simulink model "BEVModel_Alternate"  (R2023a)
settings: Solver=VariableStepAuto  StartTime=0.0  StopTime=1  RelTol=1e-3
undefined symbols (not defined in the file or in its folder): Ion, Lithium
libraries: fl_lib x9, nesl_utility x7, ee_lib x3, autolibshared x2, spsBatteryLib x1, spsControlledCurrentSourceLib x1, sps_lib x1
settings Model: Creator=koush  LastModifiedBy=koush

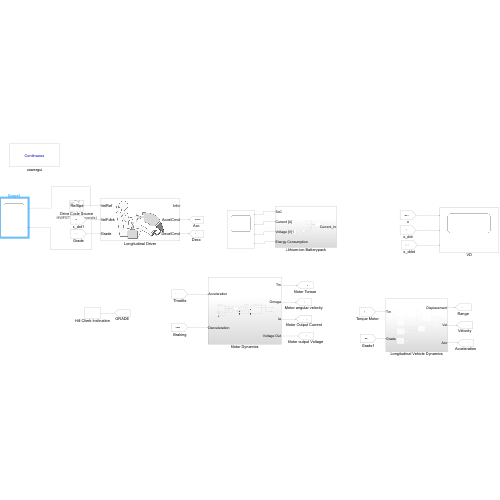
[thumbnail: Simulink's stored preview of the top-level diagram]
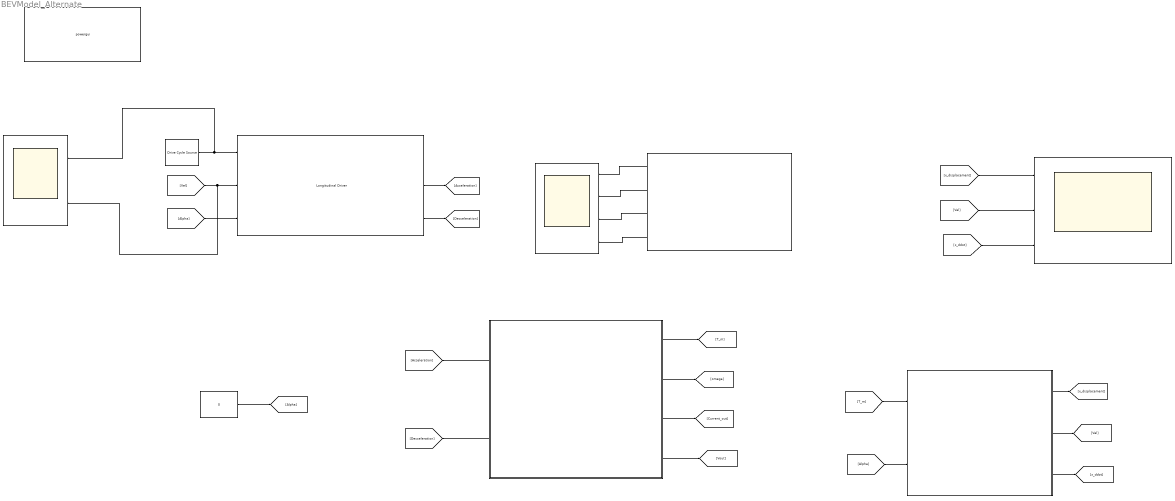
== system BEVModel_Alternate ==
  Drive Cycle Source : autolibshared/Drive Cycle Source  cycleVar=HWFET  fileVar=cycleFTP75.mat  tfinal="765  seconds"  cycleRepeat=off  outAccPort=off  outGearPort=off  gearList=No gear data  t_wot1=5  xdot_woto=0  xdot_wot1=30  t_wot2=20  xdot_wot2=0  t_wotend=30  srcUnit=m/s  outUnit=m/s  srcAccUnit=m/s/s  outAccUnit=m/s^2  dt=0  aMode=1  faultOption=off  velBnd=2  velBndUnit=mph  inUnit=m/s  timeBnd=1  failOption=off  stopSim=off  maxFaultCnt=10  maxFaultTime=2  maxTotFaultTime=15  traceOption=off  dtTrace=1  traceWindow=10  lastDCname=HWFET  lastOutUnit=mph  lastDT=0  lastTB=1  lastSB=2  forceCalcBound=off
  Hill Climb Inclination : Constant  Value=0
  Lithium-ion Batterypack : Subsystem
  Longitudinal Driver : autolibshared/Longitudinal Driver  extAccelOvr=off  extDecelOvr=off  extAccelHld=off  extDecelHld=off  extAccelZero=off  extDecelZero=off  cntrlType=PI  shftType=None  velUnits=m/s  gearOut=off  Kp=15  Ki=1  Kff=.05  Kg=.01  VehVelVec=[0 100]  KffVec=[.1 .1]  KpVec=[10 10]  KiVec=[5 5]  KgVec=[0 0]  m=1500  Kpt=3000  tau=.1  L=2  aR=200  bR=2.5  cR=.5  g=9.81  vnom=100  Kaw=.1  tauerr=.03  tauPt=2  GearInit=0  tShift=.1  pdlVec=[0.1 0.4 0.5 0.9]  upShftTbl=[-1 12.9375 26.4375 39.9375 51.18749999999999 62.4375 72.84375 83.25;-1 16.3125 29.8125 43.3125 54.5624 65.8125 76.78125 87.75;-1 19.6875 33.1875 46.68749999999999 57.9375 69.1875 80.71875 92.25;-1 33 52.5 77.25 100.5 138.75 161.875 185]  dwnShftTbl=[1 9.5625 23.0625 36.5625 47.8125 59.0625 68.90625 78.75;1 12.9375 26.4375 39.9375 51.18749999999999 62.4375 72.84375 83.25;1 16.3125 29.8125 43.3125 54.562499 65.8125 76.78125 87.75;1 19.6875 33.1875 46.68749999999999 57.9375 69.1875 80.71875 92.25]  tClutch=.5  tRev=.5  tPark=120  aMode=1  UpGearVec="[0  1  2  3  4  5  6  7]"  DownGearVec="[1  2  3  4  5  6  7  8]"
  Longitudinal Vehicle Dynamics : Subsystem
  Motor Dynamics : Subsystem
  Scope : Scope  NumInputPorts=4
  Scope1 : Scope  NumInputPorts=2
  VD : Scope  NumInputPorts=3
  powergui : sps_lib/powergui  Priority=1  SimulationMode=Continuous  SampleTime=50e-6  frequency=60  Iterations=50  frequencyindice=0  Pbase=100e6  ErrMax=1e-4  UnitsV=kV  UnitsW=MW  buscounter=0  FunctionMessages=off  echomessages=off  EnableUseOfTLC=off  CurrentSourceSwitches=off  DisableSnubberDevices=off  DisableRonSwitches=off  DisableVfSwitches=off  DisplayEquations=off  AutomaticDiscreteSolvers=off  SolverType=Tustin/Backward Euler (TBE)  Interpol=off  ExternalGateDelay=off  methode=off  Ts=100  x0status=blocks  SPID=on  SwTol=0  HookPort=off  NonlinearTolerance=1e-4  nMaxIteration=100  ContinueOnMaxIteration=off  RestoreLinks=warning  ResistiveCurrentMeasurement=off  Frange=[0:2:500]  Ylog=off  Xlog=on  ShowGrid=off  save=off  variable=ZData  structure=0  ZoomFFT=off  StartTime=0.0  cycles=1  DisplayStyle=1  fundamental=60  FreqAxis=off  MaxFrequency=1000  frequencyindicesteady=1  RmsSteady=1  display=off
  wires:
  [Vel] -> Scope1/2, Longitudinal Driver/2
  Longitudinal Driver/3 -> [Decceleration]
  [Alpha] -> Longitudinal Vehicle Dynamics/2(Grade)
  [x_displacement] -> VD/1
  Motor Dynamics/1(Tm) -> [T_m]
  [Alpha] -> Longitudinal Driver/3
  Drive Cycle Source/1 -> Scope1/1, Longitudinal Driver/1
  Longitudinal Vehicle Dynamics/1(Displacement) -> [x_displacement]
  [Vel] -> VD/2
  [x_ddot] -> VD/3
  [T_m] -> Longitudinal Vehicle Dynamics/1(Tm)
  Hill Climb Inclination/1 -> [Alpha]
  Longitudinal Vehicle Dynamics/2(Vel) -> [Vel]
  Longitudinal Driver/2 -> [Acceleration]
  Longitudinal Vehicle Dynamics/3(Acc) -> [x_ddot]
  [Acceleration] -> Motor Dynamics/1(Acceleration)
  [Decceleration] -> Motor Dynamics/2(Decceleration)
  Motor Dynamics/2(Omega) -> [omega]
  Motor Dynamics/3(Ia) -> [Current_out]
  Motor Dynamics/4(Voltage Out) -> [Vout]
  Lithium-ion Batterypack/1(SoC) -> Scope/1
  Lithium-ion Batterypack/2(Current [A]) -> Scope/2
  Lithium-ion Batterypack/3(Voltage [V]1) -> Scope/3
  Lithium-ion Batterypack/4(Energy Consumption) -> Scope/4

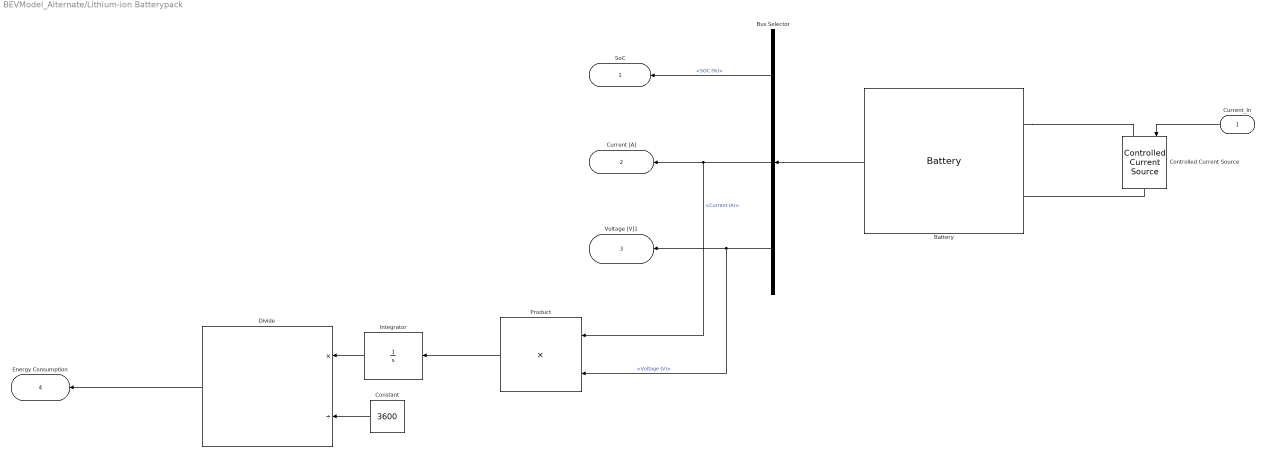
== system BEVModel_Alternate/Lithium-ion Batterypack ==
  Current_In : Inport
  Battery : spsBatteryLib/Battery  BatType=Lithium-Ion  ShowTempParam=off  ThermalPreset=no  ShowAgeParam=off  NomV=7.2  NomQ=5.4  SOC=100  Batt_Tr=30  PresetModel=on  MaxQ=5.4  MinV=5.4  FullV=8.3807  Dis_rate=2.3478  R=0.013333  Normal_OP=4.8835  expZone="[7.7788      0.2653]"  current=[6.5 13 32.5]  Units=Time  Tci=20  NomT=20  T2=-30  MaxQ2=4.8  FullV2=7.1  Normal_OP2=5.655  expZone2="[6.58           1]"  Rca=0.6  ti=2000  Dp=0  Neq0=0  Tsim=1e6  Ta1=25  Qeol=5.4*0.9  Reol=0.013333*1.2  Char_age=[2.3478, 3]  Dis_age=[2.3478, 10]  N1=1500  N2=10500  N3=1000  N4=1400  Ta2=45  N5=950
  Bus Selector : BusSelector  OutputSignals=SOC (%),Current (A),Voltage (V)
  Constant : Constant  Value=3600
  Controlled Current Source : spsControlledCurrentSourceLib/Controlled Current Source  Initialize=on  Source_Type=AC  Amplitude=0  Phase=0  Frequency=0  Measurements=None
  Divide : Product  Inputs=*/
  Integrator : Integrator
  Product : Product
  SoC : Outport
  Current [A] : Outport  Port=2
  Voltage [V]1 : Outport  Port=3
  Energy Consumption : Outport  Port=4
  wires:
  Battery/1 -> Bus Selector/1
  Current_In/1 -> Controlled Current Source/1
  Bus Selector/1 -> SoC/1  "<SOC (%)>"
  Bus Selector/2 -> Product/1, Current [A]/1  "<Current (A)>"
  Bus Selector/3 -> Product/2, Voltage [V]1/1  "<Voltage (V)>"
  Product/1 -> Integrator/1
  Integrator/1 -> Divide/1
  Constant/1 -> Divide/2
  Divide/1 -> Energy Consumption/1
  connections:
  Battery/LConn1 -- Controlled Current Source/LConn1
  Controlled Current Source/RConn1 -- Battery/LConn2

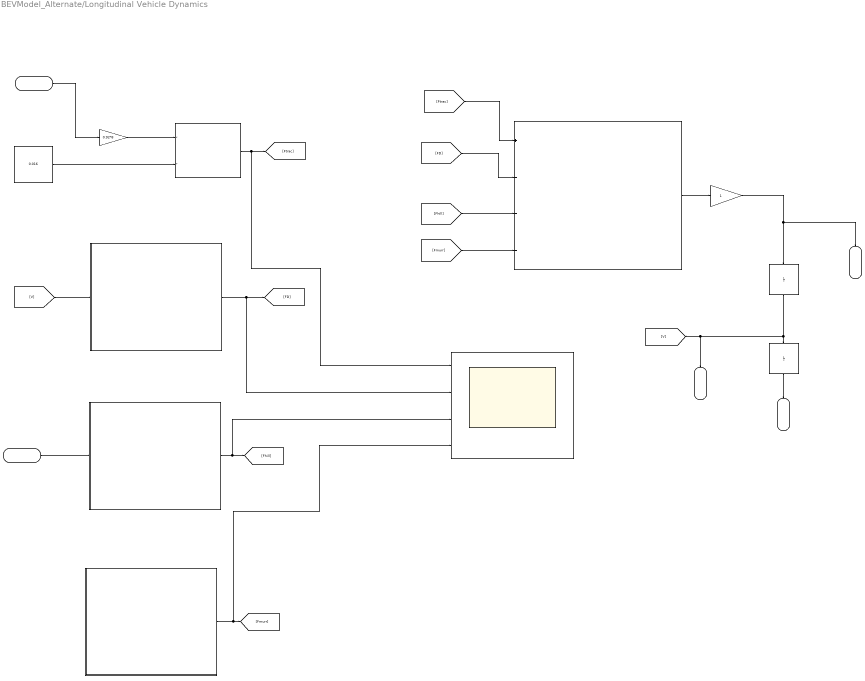
== system BEVModel_Alternate/Longitudinal Vehicle Dynamics ==
  note: Vehicle Acceleration = (Ftrac - Faero - Frr - Fhill) * (1/vehicle mass)
  Tm : Inport
  Grade : Inport  Port=2
  1/vehicle mass : Gain
  Aerodynamic Drag Force : Subsystem  TreatAsAtomicUnit=on
  Divide : Product  Inputs=*/
  Eff * Id : Gain  Gain=0.92*8
  Forces : Scope  NumInputPorts=4
  Hill Climb Force : Subsystem  TreatAsAtomicUnit=on
  Integrator : Integrator
  Integrator1 : Integrator
  Rolling Resistance Force : Subsystem  TreatAsAtomicUnit=on
  Subtract : Sum  Inputs=+---
  r_wheel : Constant  Value=0.016
  Displacement : Outport
  Vel : Outport  Port=2
  Acc : Outport  Port=3
  wires:
  Tm/1 -> Eff * Id/1  "Motor Torque"
  Eff * Id/1 -> Divide/1  "Wheel Torque"
  r_wheel/1 -> Divide/2
  [V] -> Aerodynamic Drag Force/1(Velocity)
  Aerodynamic Drag Force/1(F_drag) -> Forces/2, [FD]
  [FD] -> Subtract/2
  Divide/1 -> Forces/1, [Ftrac]  "Ftrac"
  [Ftrac] -> Subtract/1
  Grade/1 -> Hill Climb Force/1(Grade)
  Hill Climb Force/1(F_hill) -> Forces/3, [Fhill]
  [Fhill] -> Subtract/3
  Rolling Resistance Force/1(F_rr) -> Forces/4, [Fmurr]
  [Fmurr] -> Subtract/4
  Subtract/1 -> 1/vehicle mass/1
  1/vehicle mass/1 -> Acc/1, Integrator/1  "Acceleration"
  Integrator/1 -> Vel/1, [V], Integrator1/1  "Velocity"
  Integrator1/1 -> Displacement/1  "Displacement"

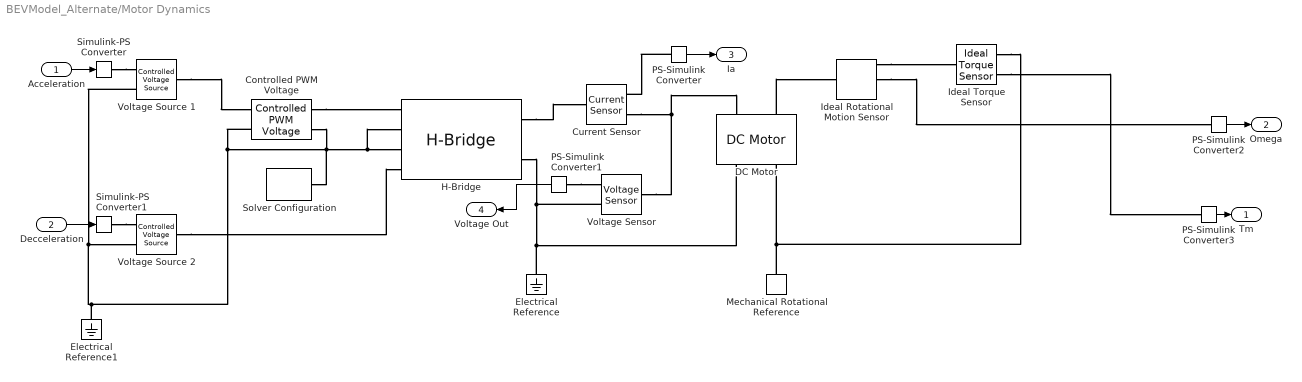
== system BEVModel_Alternate/Motor Dynamics ==
  Acceleration : Inport
  Decceleration : Inport  Port=2
  Controlled PWM Voltage : ee_lib/Integrated Circuits/Controlled PWM Voltage  F=1000 Hz  TD=0 s  pulse_width_offset=0 s  pulse_min=0 s  pwm_or_av=ee.enum.pwm_or_av.pwm  event_type=ee.enum.ic.event.asynchronous  sample_time=1e-6 s  Vmin=0 V  Vmax=5 V  Vm=5 V  u_min=0  u_max=1
  Current Sensor : fl_lib/Electrical/Electrical Sensors/Current Sensor
  DC Motor : ee_lib/Electromechanical/Brushed Motors/DC Motor  field_option=ee.enum.field_option.pm  Rf=100 Ohm  Lf=1 H  Laf=0.15 H  If0=0 A  parameterization=ee.enum.dcparam_option.circuit_param  Ra=3.9 Ohm  La=12e-6 H  emf_or_torque=ee.enum.emf_or_torque.kv  Kv=0.072e-3 V/rpm  Ki=6.876e-4 N*m/A  T_stall=0.24e-3 N*m  w_max=19100 rpm  w_rated=15000 rpm  P_rated=0.08 W  V_rated=1.5 V  lam_param=ee.enum.lam_param.damping  i_noload=0 A  V_i_noload=1.5 V  J=0.01 cm^2*g  lam=0 N*m*s/rad  speed0=0 rpm  enable_fault_armature=simscape.enum.onoff.off  rev_faulted=1 / 3  G_faulted_armature=1e-5 S  fault_trigger_armature=ee.enum.faults.faultTrigger.temporal  t_fault_armature=1 s  max_permissible_current_armature=inf A  t_fail_on_current_armature=1 s  enable_fault_field=simscape.enum.onoff.off  G_faulted_field=1e-5 S  fault_trigger_field=ee.enum.faults.faultTrigger.temporal  t_fault_field=1 s  max_permissible_current_field=inf A  t_fail_on_current_field=1 s  fault_action=simscape.enum.assert.action.none  alpha=3.93e-3 1/K  Tmeas=25 degC  thermal_mass=100 J/K  initial_temperature=25 degC
  Electrical Reference : fl_lib/Electrical/Electrical Elements/Electrical Reference
  Electrical Reference1 : fl_lib/Electrical/Electrical Elements/Electrical Reference
  H-Bridge : ee_lib/Semiconductors & Converters/Converters/H-Bridge  supply_ports=ee.enum.supply_ports.hidesupply  pwm_or_av=ee.enum.pwm_or_av.pwm  regenerative_braking_mode=ee.enum.converters.regenerative_braking_mode.depends_on_rev  discontinuous=ee.enum.current_profile.continuous  freewheeling_mode=ee.enum.converters.freewheeling_mode.one_switch_one_diode  Rload=10 Ohm  Lload=1e-5 H  F=10 kHz  Venable=2.5 V  Vmax=5.0 V  Vreverse=2.5 V  Vbrake=2.5 V  Vm=12 V  Ron=0.1 Ohm  Don=0.05 Ohm  Goff=1e-6 S  Tmeas=298.15 K  Ron2=0.1 Ohm  Don2=0.05 Ohm  Tmeas2=398.15 K  thermal_mass=100 J/K  initial_temperature=298.15 K
  Ideal Rotational Motion Sensor : fl_lib/Mechanical/Mechanical Sensors/Ideal Rotational Motion Sensor  reference=foundation.enum.MeasurementReference.difference  acceleration_port=false  velocity_port=true  position_port=true  wrap_angle=false  offset=0 rad
  Ideal Torque Sensor : fl_lib/Mechanical/Mechanical Sensors/Ideal Torque Sensor
  Mechanical Rotational Reference : fl_lib/Mechanical/Rotational Elements/Mechanical Rotational Reference
  PS-Simulink Converter{,1..3} (4 alike) : nesl_utility/PS-Simulink Converter  PhysicalDomain=network_engine_domain  SubClassName=ps_output  LeftPortType=input  RightPortType=output  PseudoPeriodic=off  Frequencies=[]  VectorFormat=inherit  Unit=inherit  AffineConversion=off
  Simulink-PS Converter : nesl_utility/Simulink-PS Converter  PhysicalDomain=network_engine_domain  SubClassName=ps_input  LeftPortType=input  RightPortType=output  PseudoPeriodic=off  Frequencies=[]  NoiseDistribution=none  NoiseParameters=[]  Unit=1  AffineConversion=off  FilteringAndDerivatives=provide  SimscapeFilterOrder=1  InputFilterTimeConstant=0.001  UdotUserProvided=0
  Simulink-PS Converter1 : nesl_utility/Simulink-PS Converter  PhysicalDomain=network_engine_domain  SubClassName=ps_input  LeftPortType=input  RightPortType=output  PseudoPeriodic=off  Frequencies=[]  NoiseDistribution=none  NoiseParameters=[]  Unit=1  AffineConversion=off  FilteringAndDerivatives=provide  SimscapeFilterOrder=1  InputFilterTimeConstant=0.001  UdotUserProvided=0
  Solver Configuration : nesl_utility/Solver Configuration  PhysicalDomain=network_engine_domain  SubClassName=solver  LeftPortType=input  RightPortType=generic  Tones=[]  Harmonics=[]  SimulateNoise=off  Profile=off  UseLocalSampling=off  EnableSwitchedLinearOptims=on  FrequencyDomain=off  UseCCode=off  RelTol=0.001  AbsTol=0.001  MinStep=1e-09  ToWorkspace=off  RevertToSquareIcSolve=off  NumHomotopyIterations=100  PhasorMode=off  PhasorModeNumHarmonics=1  ConsistencySolver=NEWTON_XTOL_AFTER_FTOL  IndexReductionMethod=DerivativeReplacement  DoDC=off  ResidualTolerance=1e-09  ConsistencyTolSource=GLOBAL  ConsistencyAbsTol=0.001  ConsistencyRelTol=0.001  ConsistencyTolFactor=0.001  UseLocalSolver=off  LocalSolverChoice=NE_BACKWARD_EULER_ADVANCER  ResolveIndetEquations=on  FunctionEvalNumThread=1  LocalSolverSampleTime=0.001  DoFixedCost=off  MaxNonlinIter=3  MaxModeIter=2  ComputeImpulses=off  ImpulseIterations=2  LinearAlgebra=auto  LinearAlgebraNumThread=0  EquationFormulation=NE_TIME_EF  DelaysMemoryBudget=1024  AutomaticFiltering=on  FilteringTimeConstant=0.001  PartitionStorageMethod=AS_NEEDED  PartitionMemoryBudget=1024  PartitionMethod=ROBUST
  Voltage Sensor : fl_lib/Electrical/Electrical Sensors/Voltage Sensor
  Voltage Source 1 : fl_lib/Electrical/Electrical Sources/Controlled Voltage Source
  Voltage Source 2 : fl_lib/Electrical/Electrical Sources/Controlled Voltage Source
  Tm : Outport
  Omega : Outport  Port=2
  Ia : Outport  Port=3
  Voltage Out : Outport  Port=4
  wires:
  PS-Simulink Converter/1 -> Ia/1
  PS-Simulink Converter1/1 -> Voltage Out/1
  Acceleration/1 -> Simulink-PS Converter/1
  Decceleration/1 -> Simulink-PS Converter1/1
  PS-Simulink Converter3/1 -> Tm/1
  PS-Simulink Converter2/1 -> Omega/1
  connections:
  H-Bridge/RConn1 -- Current Sensor/LConn1
  Current Sensor/RConn2 -- DC Motor/LConn1 -- Voltage Sensor/LConn1
  PS-Simulink Converter/LConn1 -- Current Sensor/RConn1
  H-Bridge/RConn2 -- DC Motor/RConn1 -- Electrical Reference/LConn1 -- Voltage Sensor/RConn2
  PS-Simulink Converter1/LConn1 -- Voltage Sensor/RConn1
  Controlled PWM Voltage/RConn1 -- H-Bridge/LConn1
  Simulink-PS Converter/RConn1 -- Voltage Source 1/RConn1
  Simulink-PS Converter1/RConn1 -- Voltage Source 2/RConn1
  Voltage Source 1/LConn1 -- Controlled PWM Voltage/LConn1
  Voltage Source 2/LConn1 -- H-Bridge/LConn4
  Controlled PWM Voltage/RConn2 -- Controlled PWM Voltage/LConn2 -- Voltage Source 1/RConn2 -- Voltage Source 2/RConn2 -- Electrical Reference1/LConn1 -- Solver Configuration/RConn1 -- H-Bridge/LConn2 -- H-Bridge/LConn3
  Mechanical Rotational Reference/LConn1 -- Ideal Torque Sensor/RConn1 -- DC Motor/RConn2
  DC Motor/LConn2 -- Ideal Rotational Motion Sensor/LConn1
  Ideal Rotational Motion Sensor/RConn1 -- Ideal Torque Sensor/LConn1
  Ideal Torque Sensor/RConn2 -- PS-Simulink Converter3/LConn1
  Ideal Rotational Motion Sensor/RConn2 -- PS-Simulink Converter2/LConn1

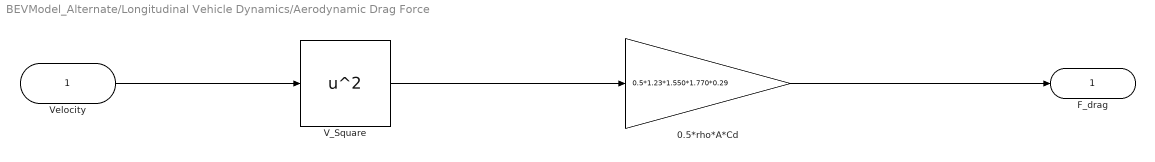
== system BEVModel_Alternate/Longitudinal Vehicle Dynamics/Aerodynamic Drag Force ==
  Velocity : Inport
  0.5*rho*A*Cd : Gain  Gain=0.5*1.23*1.550*1.770*0.29
  V_Square : Math  Operator=square
  F_drag : Outport
  wires:
  Velocity/1 -> V_Square/1
  V_Square/1 -> 0.5*rho*A*Cd/1
  0.5*rho*A*Cd/1 -> F_drag/1

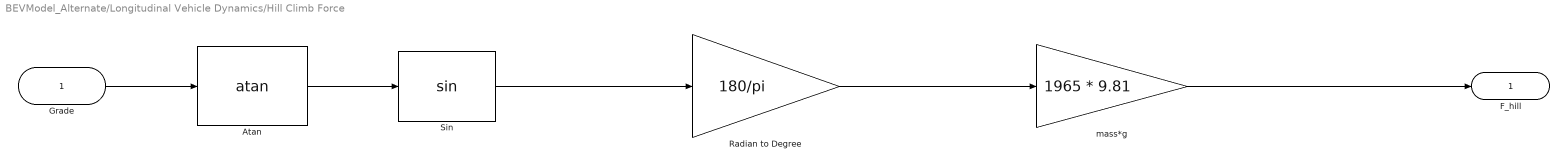
== system BEVModel_Alternate/Longitudinal Vehicle Dynamics/Hill Climb Force ==
  Grade : Inport
  Atan : Trigonometry  Operator=atan
  "Radian to Degree " : Gain  Gain=180/pi
  Sin : Trigonometry
  mass*g : Gain  Gain=1965 * 9.81
  F_hill : Outport
  wires:
  mass*g/1 -> F_hill/1
  Grade/1 -> Atan/1
  Atan/1 -> Sin/1
  Sin/1 -> "Radian to Degree "/1
  "Radian to Degree "/1 -> mass*g/1

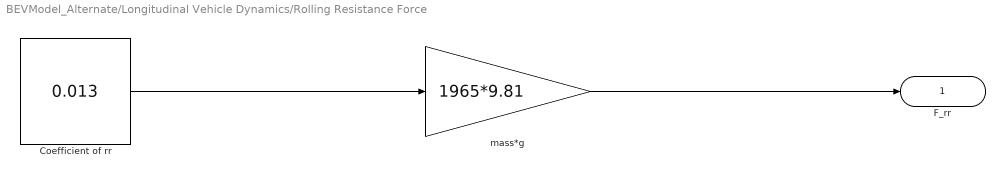
== system BEVModel_Alternate/Longitudinal Vehicle Dynamics/Rolling Resistance Force ==
  Coefficient of rr : Constant  Value=0.013
  mass*g : Gain  Gain=1965*9.81
  F_rr : Outport
  wires:
  mass*g/1 -> F_rr/1
  Coefficient of rr/1 -> mass*g/1
